simulink model "model"  (R2020b)
settings: Solver=VariableStepAuto  StartTime=0.0  StopTime=10.0  RelTol=1e-3
values from neighbouring files (symbols this model uses):
  k1 = u(1)    [f.m]    (also in h.m; runme.m = 2)
  k2 = u(2)    [f.m]    (also in h.m; runme.m = 2)
  state0 = [1;0]    [runme.m]
settings Model: Creator=fulvioforni  LastModifiedBy=fulvioforni

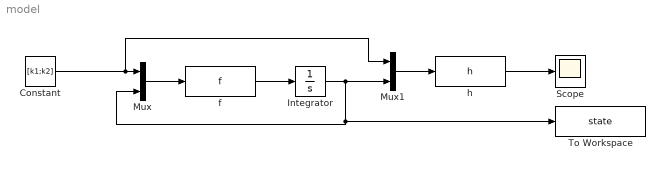
== system model ==
  Constant : Constant  Value=[k1;k2]
  Integrator : Integrator  InitialCondition=state0
  Mux : Mux  Inputs=2
  Mux1 : Mux  Inputs=2
  Scope : Scope
  To Workspace : ToWorkspace  VariableName=state  SaveFormat=Timeseries  SampleTime=-1
  f : MATLABFcn  MATLABFcn=f
  h : MATLABFcn  MATLABFcn=h
  wires:
  f/1 -> Integrator/1
  Integrator/1 -> Mux1/2, To Workspace/1, Mux/2
  Mux/1 -> f/1
  Constant/1 -> Mux1/1, Mux/1
  h/1 -> Scope/1
  Mux1/1 -> h/1
